simulink model "AERO421_FP3"  (R2024b)
settings: Solver=VariableStepAuto  StartTime=0.0  StopTime=tspan  FixedStep=10  RelTol=1e-8
model workspace (MATLAB code in the model file):
  | mu = 398601; % km
  | Re = 6378.137; %km
values from neighbouring files (symbols this model uses):
  E_b_ECI_0 = C2EulerAngles(C_b_ECI_0)    [AERO421_FP3_RJF_SR.m]
  J = [812.0396             0             0 ... (first row only)    [AERO421_FP3_RJF_SR.m]
  JD_0 = 2460390    [AERO421_FP3_RJF_SR.m]
  m_b = [0; 0; -0.5]    [AERO421_FP3_RJF_SR.m]
  q_b_ECI_0 = rotm2quat(C_b_ECI_0)    [AERO421_FP3_RJF_SR.m]
  sun_ECI = [0 0 -1]    [AERO421_FP3_RJF_SR.m]
  surfaceProperties = [Areas cps normals ... (first row only)    [AERO421_FP3_RJF_SR.m]
  T_c = [0; 0; 0]    [AERO421_FP3_RJF_SR.m]
  w_b_ECI_0 = [0.001; -0.001; 0.002]    [AERO421_FP3_RJF_SR.m]
undefined symbols (not defined in the file or in its folder): r_ECI_0, v_ECI_0
settings Model: Creator=emehiel  LastModifiedBy=rosha
settings SolverCC: AlgebraicLoopSolver=TrustRegion
settings DebuggingCC: UnconnectedInputMsg=warning  UnconnectedOutputMsg=warning  UnconnectedLineMsg=warning
settings ModelReferenceCC: EnableRefExpFcnMdlSchedulingChecks=on
settings RTWCC: GPUComputeCapability=3.5

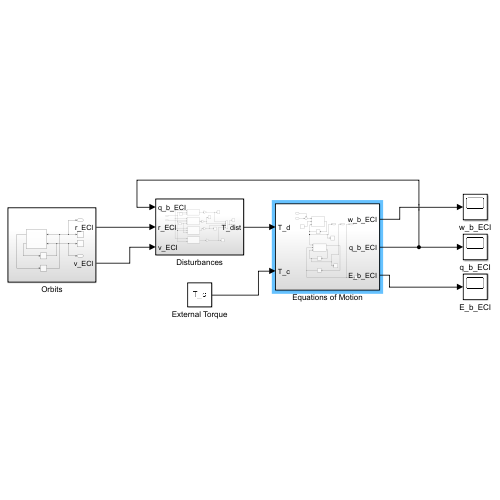
[thumbnail: Simulink's stored preview of the top-level diagram]
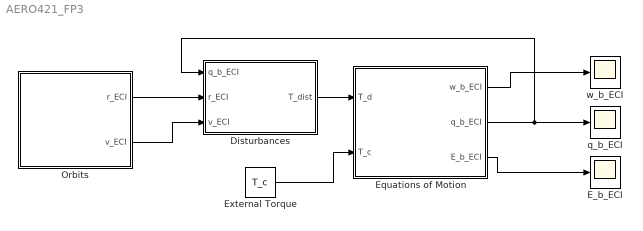
== system AERO421_FP3 ==
  Disturbances : Subsystem
  E_b_ECI : Scope
  Equations of Motion : Subsystem
  External Torque : Constant  Value=T_c
  Orbits : Subsystem
  q_b_ECI : Scope
  w_b_ECI : Scope
  wires:
  Orbits/1(r_ECI) -> Disturbances/2(r_ECI)
  Orbits/2(v_ECI) -> Disturbances/3(v_ECI)
  Equations of Motion/2(q_b_ECI) -> Disturbances/1(q_b_ECI), q_b_ECI/1
  Equations of Motion/1(w_b_ECI) -> w_b_ECI/1
  Disturbances/1(T_dist) -> Equations of Motion/1(T_d)
  Equations of Motion/3(E_b_ECI) -> E_b_ECI/1
  External Torque/1 -> Equations of Motion/2(T_c)

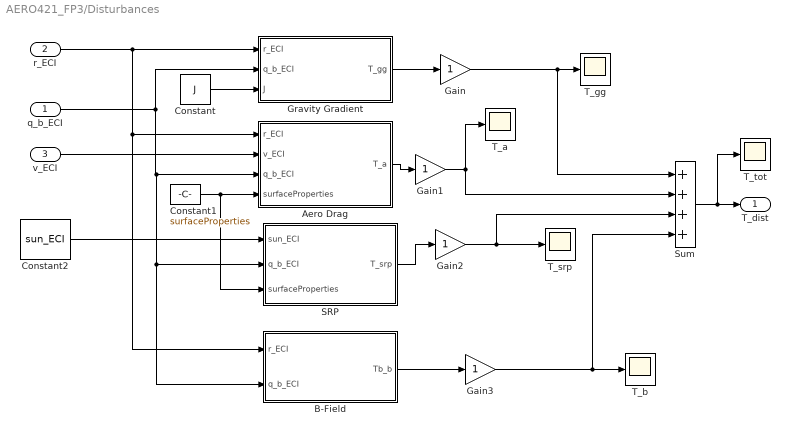
== system AERO421_FP3/Disturbances ==
  q_b_ECI : Inport
  r_ECI : Inport  Port=2
  v_ECI : Inport  Port=3
  Aero Drag : MATLAB Function  TreatAsAtomicUnit=on
  B-Field : Subsystem
  Constant : Constant  Value=J
  Constant1 : Constant  Value=surfaceProperties
  Constant2 : Constant  Value=sun_ECI
  Gain{,1..3} (4 alike) : Gain
  Gravity Gradient : MATLAB Function  TreatAsAtomicUnit=on
  SRP : MATLAB Function  TreatAsAtomicUnit=on
  Sum : Sum  Inputs=++++
  T_a : Scope
  T_b : Scope
  T_gg : Scope
  T_srp : Scope
  T_tot : Scope
  T_dist : Outport
  wires:
  Sum/1 -> T_tot/1, T_dist/1
  Aero Drag/1(T_a) -> Gain1/1
  Gravity Gradient/1(T_gg) -> Gain/1
  SRP/1(T_srp) -> Gain2/1
  Constant1/1 -> SRP/3(surfaceProperties), Aero Drag/4(surfaceProperties)
  v_ECI/1 -> Aero Drag/2(v_ECI)
  q_b_ECI/1 -> B-Field/2(q_b_ECI), SRP/2(q_b_ECI), Aero Drag/3(q_b_ECI), Gravity Gradient/2(q_b_ECI)
  Constant/1 -> Gravity Gradient/3(J)
  Constant2/1 -> SRP/1(sun_ECI)
  r_ECI/1 -> B-Field/1(r_ECI), Aero Drag/1(r_ECI), Gravity Gradient/1(r_ECI)
  B-Field/1(Tb_b) -> Gain3/1
  Gain/1 -> Sum/1, T_gg/1
  Gain1/1 -> Sum/2, T_a/1
  Gain2/1 -> Sum/3, T_srp/1
  Gain3/1 -> T_b/1, Sum/4

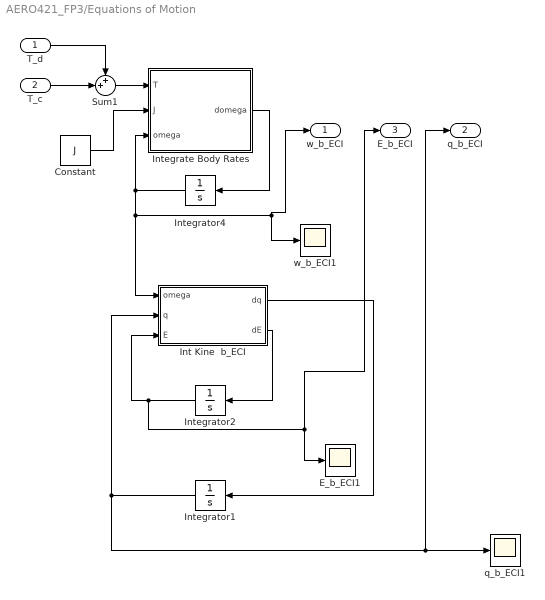
== system AERO421_FP3/Equations of Motion ==
  T_d : Inport
  T_c : Inport  Port=2
  Constant : Constant  Value=J
  E_b_ECI1 : Scope
  Int Kine  b_ECI : MATLAB Function  TreatAsAtomicUnit=on
  Integrate Body Rates : MATLAB Function  TreatAsAtomicUnit=on
  Integrator1 : Integrator  InitialCondition=q_b_ECI_0
  Integrator2 : Integrator  InitialCondition=E_b_ECI_0
  Integrator4 : Integrator  InitialCondition=w_b_ECI_0
  Sum1 : Sum  Inputs=++|
  q_b_ECI1 : Scope
  w_b_ECI1 : Scope
  w_b_ECI : Outport  VectorParamsAs1DForOutWhenUnconnected=off
  q_b_ECI : Outport  Port=2  VectorParamsAs1DForOutWhenUnconnected=off
  E_b_ECI : Outport  Port=3  VectorParamsAs1DForOutWhenUnconnected=off
  wires:
  Integrator2/1 -> E_b_ECI/1, E_b_ECI1/1, Int Kine  b_ECI/3(E)
  T_d/1 -> Sum1/1
  T_c/1 -> Sum1/2
  Integrator4/1 -> w_b_ECI1/1, w_b_ECI/1, Int Kine  b_ECI/1(omega), Integrate Body Rates/3(omega)
  Int Kine  b_ECI/1(dq) -> Integrator1/1
  Int Kine  b_ECI/2(dE) -> Integrator2/1
  Sum1/1 -> Integrate Body Rates/1(T)
  Constant/1 -> Integrate Body Rates/2(J)
  Integrate Body Rates/1(domega) -> Integrator4/1
  Integrator1/1 -> Int Kine  b_ECI/2(q), q_b_ECI1/1, q_b_ECI/1

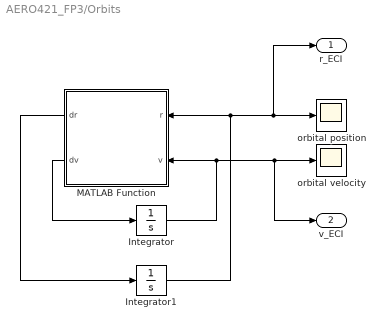
== system AERO421_FP3/Orbits ==
  Integrator : Integrator  InitialCondition=v_ECI_0
  Integrator1 : Integrator  InitialCondition=r_ECI_0
  MATLAB Function : MATLAB Function  TreatAsAtomicUnit=on
  orbital position : Scope
  orbital velocity : Scope
  r_ECI : Outport  VectorParamsAs1DForOutWhenUnconnected=off
  v_ECI : Outport  Port=2  VectorParamsAs1DForOutWhenUnconnected=off
  wires:
  Integrator/1 -> v_ECI/1, orbital velocity/1, MATLAB Function/2(v)
  Integrator1/1 -> r_ECI/1, orbital position/1, MATLAB Function/1(r)
  MATLAB Function/1(dr) -> Integrator1/1
  MATLAB Function/2(dv) -> Integrator/1

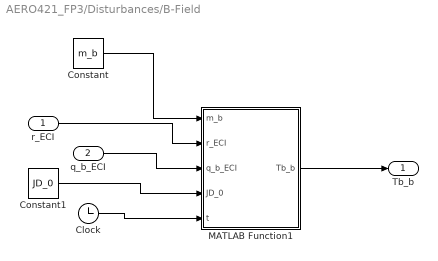
== system AERO421_FP3/Disturbances/B-Field ==
  r_ECI : Inport
  q_b_ECI : Inport  Port=2
  Clock : Clock
  Constant : Constant  Value=m_b  VectorParams1D=off
  Constant1 : Constant  Value=JD_0
  MATLAB Function1 : MATLAB Function  TreatAsAtomicUnit=on
  Tb_b : Outport
  wires:
  MATLAB Function1/1(Tb_b) -> Tb_b/1
  q_b_ECI/1 -> MATLAB Function1/3(q_b_ECI)
  r_ECI/1 -> MATLAB Function1/2(r_ECI)
  Clock/1 -> MATLAB Function1/5(t)
  Constant1/1 -> MATLAB Function1/4(JD_0)
  Constant/1 -> MATLAB Function1/1(m_b)

== matlab function AERO421_FP3/Equations of Motion/Int Kine  b_ECI ==
  data: omega input; q input; dq output; E input; dE output
function [dq,dE] = kinematics(omega, q, E)
%#codegen

% unpack quaternion

epsilon = q(1:3,1);
eta = q(4,1);

depsilon = 1/2*(eta*eye(3) + vcross(epsilon))*omega;
deta = -1/2*epsilon'*omega;

dq = [depsilon; deta];

LBI = 1/cos(E(2))*[cos(E(2)) sin(E(1))*sin(E(2))  cos(E(1))*sin(E(2));
                   0         cos(E(1))*cos(E(2)) -sin(E(1))*cos(E(2));
                   0         sin(E(1))            cos(E(1))];

dE = LBI*omega;

== matlab function AERO421_FP3/Equations of Motion/Integrate Body Rates ==
  data: T input; J input; omega input; domega output
function domega = dynamics(T, J, omega)
%#codegen

domega = J\(T - cross(omega, J*omega));

== matlab function AERO421_FP3/Disturbances/Gravity Gradient ==
  data: r_ECI input; T_gg output; q_b_ECI input; J input
function T_gg = gg_torque(r_ECI, q_b_ECI, J)
mu = 398600; % km^3/s^2

C_b_ECI = quat2dcm(q_b_ECI');
r_b = C_b_ECI * r_ECI;

T_gg = 3*mu/norm(r_ECI)^5*vcross(r_b)*J*r_b;

end

== matlab function AERO421_FP3/Disturbances/Aero Drag ==
  data: r_ECI input; v_ECI input; T_a output; q_b_ECI input; surfaceProperties input
function T_a = aero_drag_torque(r_ECI, v_ECI, q_b_ECI, surfaceProperties) 
r_ECI = r_ECI*1000; % m
v_ECI = v_ECI*1000; % m/s
% Convert v_ECI to v_b
C_b_ECI_0 = quat2dcm(q_b_ECI');
v_b = C_b_ECI_0*v_ECI;
v_hat = v_b/norm(v_b);
% Calculate density using standard exponetial decay model (or model of your
% choice)
Re = 6378*1000;
Me = 5.972e+24;
h = norm(r_ECI) - Re;
G = 6.67e-11;
k = 1.381e-23;
rho0 = 3.614e-14;
Cd = 2.2;

g = G*Me/norm(r_ECI)^2;

m = 28.964/6.022e23; % CHECK UNITS
T = - 131.21 + 0.00299*h;
H = 109*1000;
h0 = 700*1000;
rho = rho0*exp(-((h-h0)/H));
T_a = [0; 0; 0];
% P = 22.65 * exp(1.73 - .000157 * h);
% rho = P/(0.2869*(T+273.15));



% Loop through all the surfaces of the MehielSat
for i = 1:length(surfaceProperties)
    % Find wetted area
    normVect = surfaceProperties(i, 5:7);
    normVect = normVect/norm(normVect);
    cpa = surfaceProperties(i, 2:4);
    areaSurf = surfaceProperties(i, 1);
    A_wet = areaSurf*dot(normVect, v_hat);
    if A_wet > 0
        % Add to total torque from atmospheric drag
        Fdrag = -0.5*Cd*rho*norm(v_b)^2*A_wet*v_hat;
        T_a = T_a + cross(cpa', Fdrag);
    end


end

== matlab function AERO421_FP3/Disturbances/SRP ==
  data: sun_ECI input; T_srp output; q_b_ECI input; surfaceProperties input
function T_srp  = SPR_torque(sun_ECI, q_b_ECI, surfaceProperties)

p_sun = 4.5e-6; %N/m (given)
C_b_ECI_0 = quat2dcm(q_b_ECI');
sun_b = C_b_ECI_0*sun_ECI;
sun_hat = sun_b/norm(sun_b);
T_srp = [0; 0; 0];

for i = 1:length(surfaceProperties)
    % Find wetted area
    normVect = surfaceProperties(i, 5:7);
    normVect = normVect/norm(normVect);
    cpa = surfaceProperties(i, 2:4);
    areaSurf = surfaceProperties(i, 1);
    A_wet = areaSurf*dot(normVect, sun_hat);
    if A_wet > 0
        % Add to total torque from solar pressure
        F_sun = -p_sun*sun_hat*A_wet;
        T_srp = T_srp + cross(cpa', F_sun);
    end
end
end

== matlab function AERO421_FP3/Orbits/MATLAB Function ==
  data: r input; dr output; v input; dv output
function [dr,dv] = orbitalDynamics(r, v)
%#codegen

mu = 398600; % km^3/s^2
    x = r(1);
    y = r(2);
    z = r(3);
    dx = v(1); %vel
    dy = v(2); %vel
    dz = v(3); %vel
    
    %mag of pos vector
    r = norm([x y z]);
    
    %accel: !!eqs of motion!!
    ddx = -mu*x/r^3;
    ddy = -mu*y/r^3;
    ddz = -mu*z/r^3;

    dr = [dx;dy;dz];
    dv = [ddx;ddy;ddz];

== matlab function AERO421_FP3/Disturbances/B-Field/MATLAB Function1 ==
  data: m_b input; r_ECI input; q_b_ECI input; Tb_b output; JD_0 input; t input
function Tb_b = WMM(m_b, r_ECI, q_b_ECI, JD_0, t)

% Constants
omega_Earth = 7.2921150e-5; % Earth's rotation rate in rad/s
r_ECI = r_ECI*1000; %convert to meters

% Time since JD_0 (in days)
delta_JD = t / 86400; % 86400 sec/day

% Current Julian Date
JD = JD_0 + delta_JD;
pos = omega_Earth*JD;
r_ECEF = rotz(rad2deg(pos))' * r_ECI;

C_b_ECI = quat2dcm(q_b_ECI');
C_ECI_ECEF = rotz(rad2deg(pos));
C_b_ECEF = C_b_ECI * C_ECI_ECEF;

% DGRF 2020 (given)
a = 6371.2; %km
g_11 = -1450.9; %nT
h_11 = 4652.5; %nT
g_10 = -29404.8; %nT
m_ECEF = a^3*[g_11; h_11; g_10]; %nT km^3
m_ECEF = m_ECEF * 1e-9 * (1e3)^3; % convert nT to T, km^3 to m^3


m = m_ECEF;
r = r_ECEF;
B = (3*dot(m,r)*r - m*norm(r)^2) / norm(r)^5; %in ECEF
B_b = C_b_ECEF * B;

Tb_b = cross(m_b,B_b);
